simulink model "simulator"  (R2016a)
settings: Solver=ode4  StartTime=0.0  StopTime=11.670000  FixedStep=0.010000  RelTol=1e-3
model workspace (MAT data in the model file):
  Sig = Simulink.Signal
  Sig.DataType = 'auto'
  Sig.Dimensions = -1
  Sig.DimensionsMode = 'auto'
  Sig.Complexity = 'auto'
  Sig.SampleTime = -1
  Sig.SamplingMode = 'auto'
libraries: simulink x3
settings Model: Creator=combine  LastModifiedBy=rasrack
settings DataIOCC: SaveFormat=Array  SignalLogging=off  DSMLogging=off  SaveTime=off

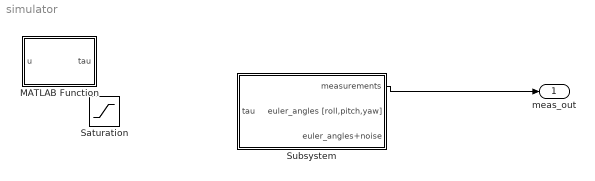
== system simulator ==
  MATLAB Function : MATLAB Function  TreatAsAtomicUnit=on
  Saturation : Saturate  UpperLimit=1  LowerLimit=-1
  Subsystem : Subsystem
  meas_out : Outport
  wires:
  Subsystem/1(measurements) -> meas_out/1

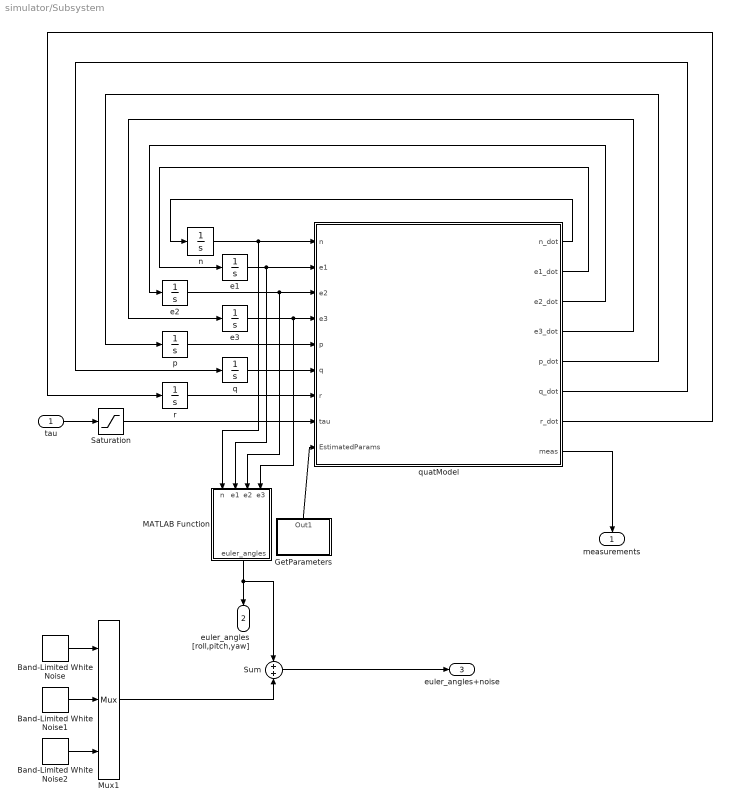
== system simulator/Subsystem ==
  tau : Inport
  Band-Limited White Noise : simulink/Sources/Band-Limited White Noise  Cov=0.0001  Ts=0.1  seed=[23341]
  Band-Limited White Noise1 : simulink/Sources/Band-Limited White Noise  Cov=0.0001  Ts=0.1  seed=[23312341]
  Band-Limited White Noise2 : simulink/Sources/Band-Limited White Noise  Cov=0.0001  Ts=0.1  seed=[2334571]
  GetParameters : Subsystem
  MATLAB Function : MATLAB Function  TreatAsAtomicUnit=on
  Mux1 : Mux  Inputs=3
  Saturation : Saturate  UpperLimit=49.9531  LowerLimit=-40.0337
  Sum : Sum  Inputs=+|+
  e1 : Integrator  InitialCondition=0.000000  ContinuousStateAttributes='e1'
  e2 : Integrator  InitialCondition=0.000000  ContinuousStateAttributes='e2'
  e3 : Integrator  InitialCondition=0.000000  ContinuousStateAttributes='e3'
  n : Integrator  InitialCondition=1.000000  ContinuousStateAttributes='n'
  p : Integrator  InitialCondition=0.000000  ContinuousStateAttributes='p'
  q : Integrator  InitialCondition=0.000000  ContinuousStateAttributes='q'
  quatModel : MATLAB Function  TreatAsAtomicUnit=on
  r : Integrator  InitialCondition=0.000000  ContinuousStateAttributes='r'
  measurements : Outport
  euler_angles [roll,pitch,yaw] : Outport  Port=2
  euler_angles+noise : Outport  Port=3  PortDimensions=7
  wires:
  quatModel/8(meas) -> measurements/1
  GetParameters/1(Out1) -> quatModel/9(EstimatedParams)
  quatModel/7(r_dot) -> r/1
  e2/1 -> quatModel/3(e2), MATLAB Function/3(e2)
  e3/1 -> quatModel/4(e3), MATLAB Function/4(e3)
  p/1 -> quatModel/5(p)
  q/1 -> quatModel/6(q)
  quatModel/1(n_dot) -> n/1
  quatModel/2(e1_dot) -> e1/1
  quatModel/5(p_dot) -> p/1
  quatModel/6(q_dot) -> q/1
  n/1 -> quatModel/1(n), MATLAB Function/1(n)
  e1/1 -> quatModel/2(e1), MATLAB Function/2(e1)
  r/1 -> quatModel/7(r)
  quatModel/3(e2_dot) -> e2/1
  quatModel/4(e3_dot) -> e3/1
  MATLAB Function/1(euler_angles) -> Sum/1, euler_angles [roll,pitch,yaw]/1
  Sum/1 -> euler_angles+noise/1
  Band-Limited White Noise/1 -> Mux1/1
  Band-Limited White Noise1/1 -> Mux1/2
  Mux1/1 -> Sum/2
  Band-Limited White Noise2/1 -> Mux1/3
  Saturation/1 -> quatModel/8(tau)
  tau/1 -> Saturation/1

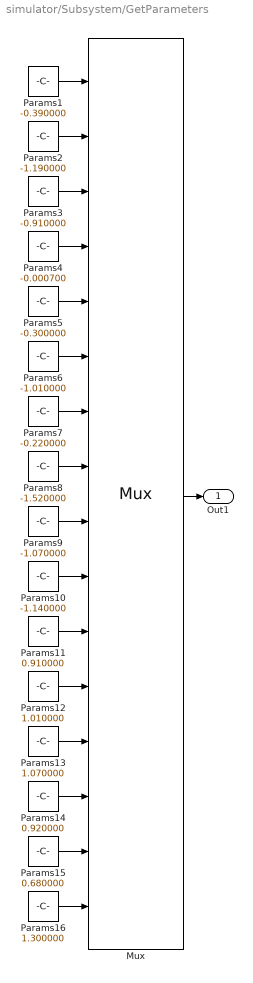
== system simulator/Subsystem/GetParameters ==
  Mux : Mux  Inputs=16
  Params1 : Constant  Value=-0.390000
  Params10 : Constant  Value=-1.140000
  Params11 : Constant  Value=0.910000
  Params12 : Constant  Value=1.010000
  Params13 : Constant  Value=1.070000
  Params14 : Constant  Value=0.920000
  Params15 : Constant  Value=0.680000
  Params16 : Constant  Value=1.300000
  Params2 : Constant  Value=-1.190000
  Params3 : Constant  Value=-0.910000
  Params4 : Constant  Value=-0.000700
  Params5 : Constant  Value=-0.300000
  Params6 : Constant  Value=-1.010000
  Params7 : Constant  Value=-0.220000
  Params8 : Constant  Value=-1.520000
  Params9 : Constant  Value=-1.070000
  Out1 : Outport
  wires:
  Params10/1 -> Mux/10
  Params14/1 -> Mux/14
  Params1/1 -> Mux/1
  Params16/1 -> Mux/16
  Params11/1 -> Mux/11
  Params13/1 -> Mux/13
  Params5/1 -> Mux/5
  Params4/1 -> Mux/4
  Params9/1 -> Mux/9
  Params15/1 -> Mux/15
  Mux/1 -> Out1/1
  Params2/1 -> Mux/2
  Params3/1 -> Mux/3
  Params8/1 -> Mux/8
  Params7/1 -> Mux/7
  Params6/1 -> Mux/6
  Params12/1 -> Mux/12

== matlab function simulator/Subsystem/MATLAB Function ==
  data: n input; euler_angles output; e1 input; e2 input; e3 input
function euler_angles = fcn(n, e1, e2,e3)
%#codegen
  roll = atan2(n*e1*2.0+e2*e3*2.0,(e1*e1)*-2.0-(e2*e2)*2.0+1.0);
  pitch = -asin(n*e2*-2.0+e1*e3*2.0);
  yaw = atan2(n*e3*2.0+e1*e2*2.0,(e2*e2)*-2.0-(e3*e3)*2.0+1.0);

  roll = mod(roll + pi,2.0*pi) - pi;
  pitch= mod(pitch + pi,2.0*pi) - pi;
  yaw = mod(yaw + pi,2.0*pi) - pi;

euler_angles = [roll, pitch, yaw];

== matlab function simulator/Subsystem/quatModel ==
  data: n input; n_dot output; e1 input; e2 input; e3 input; p input; q input; r input; tau input size=6; e1_dot output; e2_dot output; e3_dot output; p_dot output; q_dot output; r_dot output; EstimatedParams input; meas output
function [n_dot,e1_dot,e2_dot,e3_dot,p_dot,q_dot,r_dot,meas] = quatModel(n,e1,e2,e3,p,q,r,tau,EstimatedParams)
%#codegen
m=6.621;%ROVmass[kg];
g=9.81744;%Gravity[m/s^2]
rho=1000;%waterdensity[kg/m^3]
V=0.012;%Discplacedwatervolume[m^3]
%ThrusterplacementfromCO[m]
lx1=0.16;
ly1=0.11;
ly2=0.11;
lx2=0.16;
ly3=0.11;
lx5=0.2;
ly4=0.11;
lz6=0.11;
B=m*g;
%extractforcesfromthrusters
f1=tau(1);
f2=tau(2);
f3=tau(3);
f4=tau(4);
f5=tau(5);
f6=tau(6);
g = 9.81744;


zb          = EstimatedParams(1);
Kp          = EstimatedParams(2);
Kp_dot      = EstimatedParams(3);
Kp_abs_p    = EstimatedParams(4); 
Mq          = EstimatedParams(5);
Mq_dot      = EstimatedParams(6);
Mq_abs_q    = EstimatedParams(7);
Nr          = EstimatedParams(8);
Nr_dot      = EstimatedParams(9);
Nr_abs_r    = EstimatedParams(10);
Ix          = EstimatedParams(11);
Iy          = EstimatedParams(12);
Iz          = EstimatedParams(13);
Ix_Kp_dot   = EstimatedParams(14);
Iy_Mq_dot   = EstimatedParams(15);
Iz_Nr_dot   = EstimatedParams(16);

mag_n= 10;
mag_e=10;
mag_d=10;
n_dot=- (e1*p)/2 - (e2*q)/2 - (e3*r)/2 - n*(50*e1^2 + 50*e2^2 + 50*e3^2 + 50*n^2 - 50);
e1_dot=   (e2*r)/2 - (e3*q)/2 + (n*p)/2 - e1*(50*e1^2 + 50*e2^2 + 50*e3^2 + 50*n^2 - 50);
e2_dot=   (e3*p)/2 - (e1*r)/2 + (n*q)/2 - e2*(50*e1^2 + 50*e2^2 + 50*e3^2 + 50*n^2 - 50);
e3_dot=   (e1*q)/2 - (e2*p)/2 + (n*r)/2 - e3*(50*e1^2 + 50*e2^2 + 50*e3^2 + 50*n^2 - 50);
p_dot=(f1*ly1-f2*ly2+f6*lz6+p*(Kp+Kp_abs_p*abs(p))-Mq_dot*q*r+Nr_dot*q*r+q*r*(Iy-Iz)+B*zb*(2*e2*e3+2*e1*n))/Ix_Kp_dot;
q_dot=(f1*lx1+f2*lx2-f5*lx5+q*(Mq+Mq_abs_q*abs(q))+Kp_dot*p*r-Nr_dot*p*r-p*r*(Ix-Iz)-B*zb*(2*e1*e3-2*e2*n))/Iy_Mq_dot;
r_dot=(r*(Nr+Nr_abs_r*abs(r))+f3*ly3-f4*ly4-Kp_dot*p*q+Mq_dot*p*q+p*q*(Ix-Iy))/Iz_Nr_dot;

meas=zeros(9,1);
meas(1) = p; 
meas(2) = q;
meas(3) = r;
meas(4) =-g*(2*e1*e3 - 2*e2*n);
meas(5) = -g*(2*e2*e3 + 2*e1*n);
meas(6) = g*(2*e1^2 + 2*e2^2 - 1);
meas(7) = mag_d*(2*e1*e3 - 2*e2*n) - (mag_e^2 + mag_n^2)^(1/2)*(2*e2^2 + 2*e3^2 - 1);
meas(8) = (2*e1*e2 - 2*e3*n)*(mag_e^2 + mag_n^2)^(1/2) + mag_d*(2*e2*e3 + 2*e1*n);
meas(9) = (2*e1*e3 + 2*e2*n)*(mag_e^2 + mag_n^2)^(1/2) - mag_d*(2*e1^2 + 2*e2^2 - 1);

== matlab function simulator/MATLAB Function ==
  data: u input; tau output
function tau = fcn(u)
%#codegen
lookup =[...
    -40.0337   -1.0000
    -40.0337   -0.9750
    -40.0788   -0.9500
    -37.5428   -0.9250
    -36.6092   -0.9000
    -35.4971   -0.8750
    -33.7623   -0.8500
    -32.3835   -0.8250
    -31.2263   -0.8000
    -29.9809   -0.7750
    -28.5128   -0.7500
    -27.6234   -0.7250
    -26.5554   -0.7000
    -24.7765   -0.6750
    -23.1751   -0.6500
    -22.1522   -0.6250
    -21.3510   -0.6000
    -19.5280   -0.5750
    -18.4600   -0.5500
    -17.3480   -0.5250
    -16.1025   -0.5000
    -14.6345   -0.4750
    -13.0781   -0.4500
    -12.1877   -0.4250
    -10.9874   -0.4000
    -10.0528   -0.3750
    -8.8966   -0.3500
    -7.7404   -0.3250
    -6.8058   -0.3000
    -6.0497   -0.2750
    -5.1151   -0.2500
    -4.2698   -0.2250
    -3.4696   -0.2000
    -2.7135   -0.1750
    -1.8682   -0.1500
    -1.1121   -0.1250
    -0.5335   -0.1000
    -0.2667   -0.0750
    0   -0.0500
    0   -0.0250
    0         0
    0    0.0250
    0    0.0500
    0.5786    0.0750
    1.1121    0.1000
    1.8240    0.1250
    2.5801    0.1500
    3.4255    0.1750
    4.0923    0.2000
    5.1151    0.2250
    6.2272    0.2500
    7.0284    0.2750
    8.2739    0.3000
    9.2526    0.3250
    10.8089    0.3500
    12.2328    0.3750
    13.6558    0.4000
    14.9904    0.4250
    16.4585    0.4500
    17.7039    0.4750
    19.2161    0.5000
    20.5508    0.5250
    21.7521    0.5500
    23.6644    0.5750
    24.7324    0.6000
    26.4221    0.6250
    27.7126    0.6500
    29.6249    0.6750
    31.3156    0.7000
    32.8729    0.7250
    33.8065    0.7500
    34.2517    0.7750
    37.0534    0.8000
    38.6549    0.8250
    39.2776    0.8500
    41.1458    0.8750
    42.9257    0.9000
    44.7938    0.9250
    47.1062    0.9500
    48.0408    0.9750
    49.9531    1.0000];
%Thrustherforce in newtons.
tau(1) = interp1(lookup(:,2),lookup(:,1),u(1));
tau(2) = interp1(lookup(:,2),lookup(:,1),u(2));
tau(3) = interp1(lookup(:,2),lookup(:,1),u(3));
tau(4) = interp1(lookup(:,2),lookup(:,1),u(4));
tau(5) = interp1(lookup(:,2),lookup(:,1),u(5));
tau(6) = interp1(lookup(:,2),lookup(:,1),u(6));

end
